simulink model "sl_arm_ibvs"  (Simulink 8.4)
settings: Solver=ode45  StartTime=0.0  StopTime=20.0  RelTol=1e-3
InitFcn:
  | mdl_puma560
  | camera = CentralCamera('default');
  | P = mkgrid(2, 0.5, troty(pi/2)*transl(0,0,2.5));
  | q0 = [0 pi/4 pi 0 pi/4 -pi/4]';
libraries: roblocks x7
settings Model: Creator=pic  LastModifiedBy=corkep  ExtModeTrigMode=oneshot  ExtModeArmWhenConnect=off
settings DataIOCC: LimitDataPoints=off  SaveFormat=StructureWithTime  ReturnWorkspaceOutputs=on
settings OptimizationCC: BlockReduction=off  BooleanDataType=off  InitFltsAndDblsToZero=on
settings DebuggingCC: SaveWithParameterizedLinksMsg=none  SignalResolutionControl=TryResolveAllWithWarning  SolverPrmCheckMsg=none  MultiTaskDSMMsg=warning  MultiTaskCondExecSysMsg=none
settings HardwareCC: TargetUnknown=on
settings RTWCC: IncludeERTFirstTime=on
settings GRTTargetCC: ModelReferenceCompliant=off  CompOptLevelCompliant=off  MatFileLogging=off

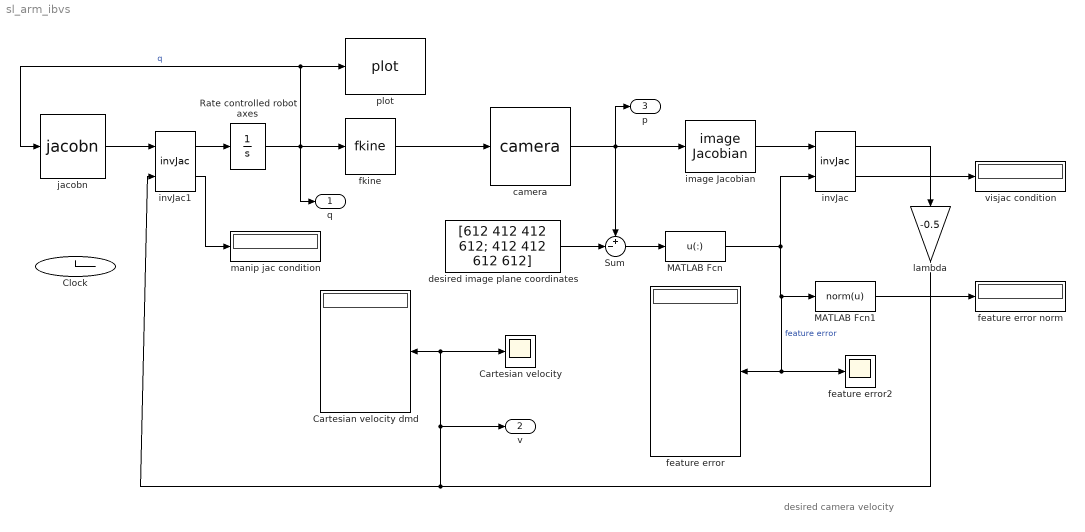
== system sl_arm_ibvs ==
  note: desired camera velocity
  Cartesian velocity : Scope
      settings: TimeRange=20  YMin=-0.4  YMax=1.9
  Cartesian velocity dmd : Display
      settings: Format=bank
  Clock : Clock
  MATLAB Fcn : MATLABFcn  MATLABFcn=u(:)  Output1D=off
  MATLAB Fcn1 : MATLABFcn  MATLABFcn=norm(u)
  Rate controlled robot axes : Integrator  InitialCondition=q0
  Sum : Sum  Inputs=+-|  SaturateOnIntegerOverflow=on  InputSameDT=on  OutDataTypeStr=Inherit: Same as first input
  camera : roblocks/Vision/camera  cam=camera  points=P
  desired image plane coordinates : Constant  Value=[612 412 412 612; 412 412 612 612]  VectorParams1D=off
  feature error : Display
      settings: Format=bank
  feature error norm : Display
  feature error2 : Scope
      settings: TimeRange=20  YMin=-150  YMax=150
  fkine : roblocks/Kinematics/fkine  robot=p560
  image Jacobian : roblocks/Vision/image Jacobian  cam=camera  z=2
  invJac : roblocks/Vision/invJac
  invJac1 : roblocks/Vision/invJac
  jacobn : roblocks/Kinematics/jacobn  robot=p560
  lambda : Gain  Gain=-0.5  SaturateOnIntegerOverflow=on  OutDataTypeStr=Inherit: Same as input  ParamDataTypeStr=Inherit: Same as input
  manip jac condition : Display
  plot : roblocks/Robot Graphics/plot  robot=p560  fps=25  holdplot=on
  visjac condition : Display
  q : Outport
  v : Outport  Port=2
  p : Outport  Port=3
  wires:
  Rate controlled robot axes/1 -> fkine/1, q/1, jacobn/1, plot/1  "q"
  jacobn/1 -> invJac1/1
  invJac1/1 -> Rate controlled robot axes/1
  fkine/1 -> camera/1
  camera/1 -> Sum/1, p/1, image Jacobian/1
  Sum/1 -> MATLAB Fcn/1
  desired image plane coordinates/1 -> Sum/2
  MATLAB Fcn/1 -> MATLAB Fcn1/1, feature error2/1, feature error/1, invJac/2  "feature error"
  invJac/2 -> visjac condition/1
  MATLAB Fcn1/1 -> feature error norm/1
  invJac/1 -> lambda/1
  image Jacobian/1 -> invJac/1
  lambda/1 -> Cartesian velocity dmd/1, Cartesian velocity/1, v/1, invJac1/2
  invJac1/2 -> manip jac condition/1
